simulink model "LAB1"  (R2023b)
settings: Solver=ode23tb  StartTime=0.0  StopTime=0.04  MaxStep=1/10000/200  RelTol=1e-3  AbsTol=1e-3
libraries: spsSeriesRLCBranchLib x4, spsCurrentMeasurementLib x3, spsVoltageMeasurementLib x3, spsMeanLib x2, spsDiodeLib x1, spsMosfetLib x1, spsDCVoltageSourceLib x1, spspowerguiLib x1
settings Model: Creator=rafae  LastModifiedBy=rafae

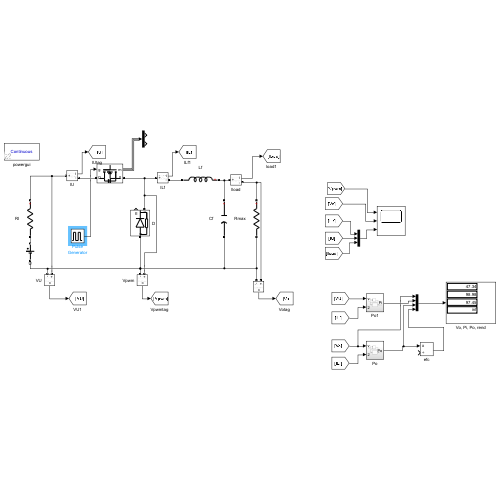
[thumbnail: Simulink's stored preview of the top-level diagram]
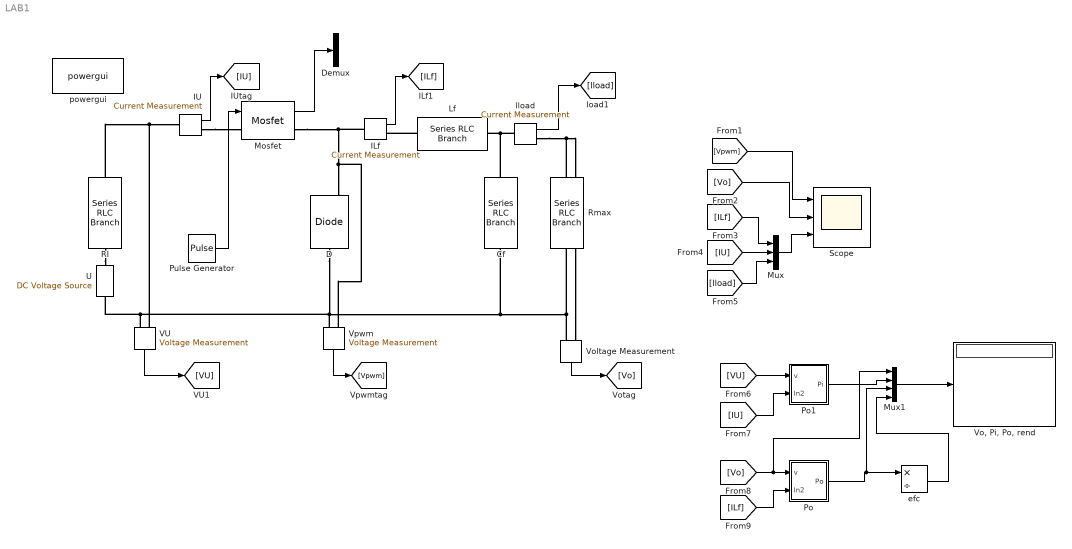
== system LAB1 ==
  Cf : spsSeriesRLCBranchLib/Series RLC Branch  LConnTagsString=__new0  RConnTagsString=__new0  BranchType=C  Resistance=1  Inductance=0  SetiL0=off  InitialCurrent=0  Capacitance=5.42e-05  Setx0=off  InitialVoltage=0  Measurements=None
  D : spsDiodeLib/Diode  Ron=0.1  Lon=0  Vf=0.8  IC=0  UseSnubber=0  Rs=10000  Cs=1e-07  Measurements=on
  Demux : Demux  Outputs=2
  ILf : spsCurrentMeasurementLib/Current Measurement  PhasorSimulation=off  OutputType=Complex  PSBequivalent=0
  IU : spsCurrentMeasurementLib/Current Measurement  PhasorSimulation=off  OutputType=Complex  PSBequivalent=0
  Lf : spsSeriesRLCBranchLib/Series RLC Branch  LConnTagsString=__new0  RConnTagsString=__new0  BranchType=L  Resistance=1  Inductance=6.78e-04  SetiL0=off  InitialCurrent=0  Capacitance=0  Setx0=off  InitialVoltage=0  Measurements=None
  Mosfet : spsMosfetLib/Mosfet  Ron=0.1  Lon=0  Rd=0.1  Vfd=0.8  IC=0  Rs=1e5  Cs=inf  Measurements=on
  Mux : Mux  Inputs=3
  Mux1 : Mux
  Po : Subsystem
  Po1 : Subsystem
  Pulse Generator : DiscretePulseGenerator  PulseType=Time based  Period=1/10000  PulseWidth=48
  RI : spsSeriesRLCBranchLib/Series RLC Branch  LConnTagsString=__new0  RConnTagsString=__new0  BranchType=R  Resistance=0.01  Inductance=0  SetiL0=off  InitialCurrent=0  Capacitance=0  Setx0=off  InitialVoltage=0  Measurements=None
  Rmax : spsSeriesRLCBranchLib/Series RLC Branch  LConnTagsString=__new0  RConnTagsString=__new0  BranchType=R  Resistance=23.04  Inductance=0  SetiL0=off  InitialCurrent=0  Capacitance=0  Setx0=off  InitialVoltage=0  Measurements=None
  Scope : Scope  NumInputPorts=3
  U : spsDCVoltageSourceLib/DC Voltage Source  Amplitude=100  Measurements=None
  VU : spsVoltageMeasurementLib/Voltage Measurement  PhasorSimulation=off  OutputType=Complex  PSBequivalent=0
  "Vo, Pi, Po, rend" : Display
  Voltage Measurement : spsVoltageMeasurementLib/Voltage Measurement  PhasorSimulation=off  OutputType=Complex  PSBequivalent=0
  Vpwm : spsVoltageMeasurementLib/Voltage Measurement  PhasorSimulation=off  OutputType=Complex  PSBequivalent=0
  efc : Product  Inputs=*/
  lload : spsCurrentMeasurementLib/Current Measurement  PhasorSimulation=off  OutputType=Complex  PSBequivalent=0
  powergui : spspowerguiLib/powergui  Priority=1  SimulationMode=Continuous  SampleTime=50e-6  frequency=60  Iterations=50  frequencyindice=0  Pbase=100e6  ErrMax=1e-4  UnitsV=kV  UnitsW=MW  buscounter=0  FunctionMessages=off  echomessages=off  EnableUseOfTLC=off  CurrentSourceSwitches=off  DisableSnubberDevices=off  DisableRonSwitches=off  DisableVfSwitches=off  DisplayEquations=off  AutomaticDiscreteSolvers=off  SolverType=Tustin/Backward Euler (TBE)  Interpol=off  ExternalGateDelay=off  methode=off  Ts=100  x0status=blocks  SPID=on  SwTol=0  HookPort=off  NonlinearTolerance=1e-4  nMaxIteration=100  ContinueOnMaxIteration=off  RestoreLinks=warning  ResistiveCurrentMeasurement=off  Frange=[0:2:500]  Ylog=off  Xlog=on  ShowGrid=off  save=off  variable=ZData  structure=0  ZoomFFT=off  StartTime=0.0  cycles=1  DisplayStyle=1  fundamental=60  FreqAxis=off  MaxFrequency=1000  frequencyindicesteady=1  RmsSteady=1  display=off
  wires:
  Pulse Generator/1 -> Mosfet/1
  VU/1 -> [VU]
  Vpwm/1 -> [Vpwm]
  Voltage Measurement/1 -> [Vo]
  lload/1 -> [lload]
  ILf/1 -> [ILf]
  IU/1 -> [IU]
  Mosfet/1 -> Demux/1
  [Vpwm] -> Scope/1
  [ILf] -> Mux/1
  [IU] -> Mux/2
  [lload] -> Mux/3
  Mux/1 -> Scope/3
  [Vo] -> Scope/2
  [VU] -> Po1/1(v)
  [IU] -> Po1/2(In2)
  [Vo] -> Mux1/1, Po/1(v)
  [ILf] -> Po/2(In2)
  Po1/1(Pi) -> Mux1/2
  efc/1 -> Mux1/4
  Po/1(Po) -> Mux1/3, efc/1
  Mux1/1 -> "Vo, Pi, Po, rend"/1
  connections:
  RI/RConn1 -- U/RConn1
  RI/LConn1 -- VU/LConn1 -- IU/LConn1
  IU/RConn1 -- Mosfet/LConn1
  Mosfet/RConn1 -- ILf/LConn1 -- Vpwm/LConn1 -- D/RConn1
  Lf/RConn1 -- ILf/RConn1
  lload/LConn1 -- Cf/LConn1 -- Lf/LConn1
  lload/RConn1 -- Voltage Measurement/LConn1 -- Rmax/LConn1
  VU/LConn2 -- D/LConn1 -- Voltage Measurement/LConn2 -- Rmax/RConn1 -- Cf/RConn1 -- Vpwm/LConn2 -- U/LConn1

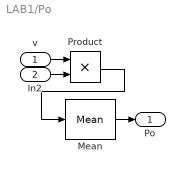
== system LAB1/Po ==
  v : Inport
  In2 : Inport  Port=2
  Mean : spsMeanLib/Mean  Freq=60  Vinit=0  Ts=0
  Product : Product
  Po : Outport
  wires:
  Mean/1 -> Po/1
  Product/1 -> Mean/1
  v/1 -> Product/1
  In2/1 -> Product/2

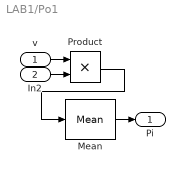
== system LAB1/Po1 ==
  v : Inport
  In2 : Inport  Port=2
  Mean : spsMeanLib/Mean  Freq=60  Vinit=0  Ts=0
  Product : Product
  Pi : Outport
  wires:
  Mean/1 -> Pi/1
  Product/1 -> Mean/1
  v/1 -> Product/1
  In2/1 -> Product/2
